simulink model "m1"  (R2020a)
settings: Solver=FixedStepAuto  StartTime=0.0  StopTime=25000.0  FixedStep=1  RelTol=1e-3
libraries: dspstat3 x12, simulink x2
settings Model: Creator=Kalev  LastModifiedBy=Kalev
settings OptimizationCC: ZeroExternalMemoryAtStartup=off  ZeroInternalMemoryAtStartup=off
settings HardwareCC: ProdBitPerPointer=32  ProdBitPerSizeT=32  ProdBitPerPtrDiffT=32  ProdLargestAtomicInteger=Long  ProdWordSize=32  ProdHWDeviceType=ARM Compatible->ARM 10
settings RTWCC: GenCodeOnly=on  TargetLang=C++
settings GRTTargetCC: TargetLangStandard=C++03 (ISO)  MultiInstanceERTCode=on  CodeInterfacePackaging=C++ class  RTWCAPIParams=on  RTWCAPIStates=on  MultiInstanceErrorCode=Warning

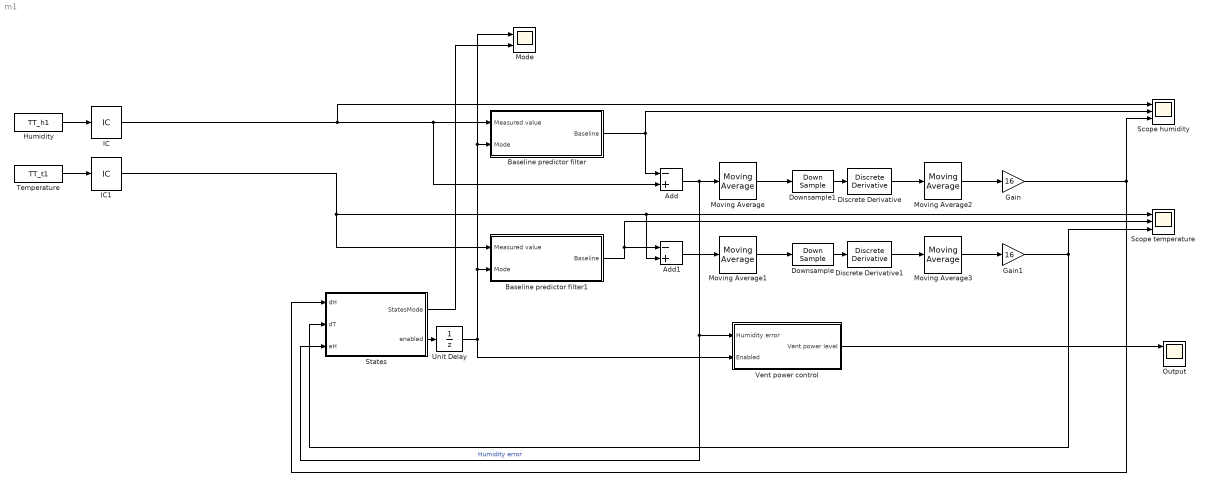
== system m1 ==
  Add : Sum  Inputs=-+
  Add1 : Sum  Inputs=-+
  Baseline predictor filter : Subsystem
  Baseline predictor filter1 : Subsystem
  Discrete Derivative : simulink/Discrete/Discrete Derivative  gainval=1.0  ICPrevScaledInput=initial_h  OutMin=[]  OutMax=[]  OutDataType=fixdt(1, 16)  OutScaling=2^-10  DoSatur=off
  Discrete Derivative1 : simulink/Discrete/Discrete Derivative  gainval=1.0  ICPrevScaledInput=initial_t  OutMin=[]  OutMax=[]  OutDataType=fixdt(1, 16)  OutScaling=2^-10  DoSatur=off
  Downsample : DownSample  N=16  phase=15  ic=initial_t
  Downsample1 : DownSample  N=16  phase=15  ic=initial_h
  Gain : Gain  Gain=16
  Gain1 : Gain  Gain=16
  Humidity : FromWorkspace  VariableName=TT_h1  OutDataTypeStr=double  SampleTime=-1
  IC : InitialCondition  Value=50
  IC1 : InitialCondition  Value=25
  Mode : Scope  NumInputPorts=2
  Moving Average{,1..3} (4 alike) : dspstat3/Moving Average  Method=Sliding window  ForgettingFactorPort=off  SpecifyWindowLength=on  WindowLength=16  ForgettingFactor=0.9  SimulateUsing=Code generation
  Output : Scope  NumInputPorts=3
  Scope humidity : Scope  NumInputPorts=3
  Scope temperature : Scope  NumInputPorts=3
  States : Stateflow chart  TreatAsAtomicUnit=on
  Temperature : FromWorkspace  VariableName=TT_t1  OutDataTypeStr=double  SampleTime=-1  OutputAfterFinalValue=Holding final value
  Unit Delay : UnitDelay  SampleTime=-1  HasFrameUpgradeWarning=on
  Vent power control : Subsystem
  wires:
  Humidity/1 -> IC/1
  Baseline predictor filter/1(Baseline) -> Scope humidity/2, Add/1
  Add/1 -> Vent power control/1(Humidity error), States/3(eH), Moving Average/1  "Humidity error"
  Temperature/1 -> IC1/1
  Add1/1 -> Moving Average1/1
  Discrete Derivative1/1 -> Moving Average3/1
  States/2(enabled) -> Unit Delay/1
  Unit Delay/1 -> Vent power control/2(Enabled), Baseline predictor filter1/2(Mode), Baseline predictor filter/2(Mode), Mode/1
  Downsample/1 -> Discrete Derivative1/1
  Downsample1/1 -> Discrete Derivative/1
  Baseline predictor filter1/1(Baseline) -> Add1/1, Scope temperature/2
  IC/1 -> Add/2, Baseline predictor filter/1(Measured value), Scope humidity/1
  IC1/1 -> Baseline predictor filter1/1(Measured value), Scope temperature/1, Add1/2
  Discrete Derivative/1 -> Moving Average2/1
  Moving Average/1 -> Downsample1/1
  Moving Average1/1 -> Downsample/1
  States/1(StatesMode) -> Mode/2
  Moving Average2/1 -> Gain/1
  Moving Average3/1 -> Gain1/1
  Gain/1 -> Scope humidity/3, States/1(dH)
  Gain1/1 -> Scope temperature/3, States/2(dT)
  Vent power control/1(Vent power level) -> Output/1

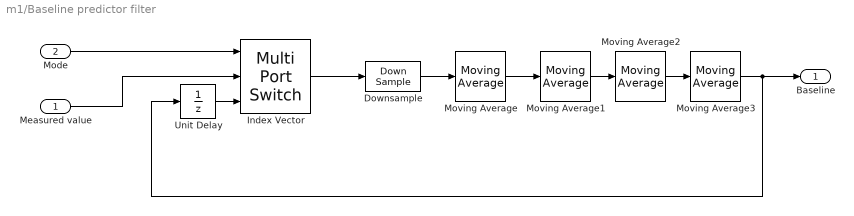
== system m1/Baseline predictor filter ==
  Measured value : Inport
  Mode : Inport  Port=2
  Downsample : DownSample  N=128
  Index Vector : MultiPortSwitch  DataPortOrder=Zero-based contiguous  Inputs=2  zeroidx=on
  Moving Average{,1..3} (4 alike) : dspstat3/Moving Average  Method=Sliding window  ForgettingFactorPort=off  SpecifyWindowLength=on  WindowLength=512  ForgettingFactor=0.9  SimulateUsing=Code generation
  Unit Delay : UnitDelay  SampleTime=-1  HasFrameUpgradeWarning=on
  Baseline : Outport
  wires:
  Moving Average1/1 -> Moving Average2/1
  Moving Average/1 -> Moving Average1/1
  Downsample/1 -> Moving Average/1
  Moving Average2/1 -> Moving Average3/1
  Index Vector/1 -> Downsample/1
  Mode/1 -> Index Vector/1
  Measured value/1 -> Index Vector/2
  Moving Average3/1 -> Unit Delay/1, Baseline/1
  Unit Delay/1 -> Index Vector/3

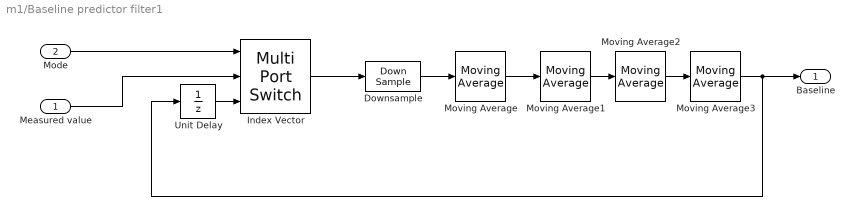
== system m1/Baseline predictor filter1 ==
  Measured value : Inport
  Mode : Inport  Port=2
  Downsample : DownSample  N=128
  Index Vector : MultiPortSwitch  DataPortOrder=Zero-based contiguous  Inputs=2  zeroidx=on
  Moving Average{,1..3} (4 alike) : dspstat3/Moving Average  Method=Sliding window  ForgettingFactorPort=off  SpecifyWindowLength=on  WindowLength=512  ForgettingFactor=0.9  SimulateUsing=Code generation
  Unit Delay : UnitDelay  SampleTime=-1  HasFrameUpgradeWarning=on
  Baseline : Outport
  wires:
  Unit Delay/1 -> Index Vector/3
  Index Vector/1 -> Downsample/1
  Moving Average3/1 -> Unit Delay/1, Baseline/1
  Measured value/1 -> Index Vector/2
  Mode/1 -> Index Vector/1
  Downsample/1 -> Moving Average/1
  Moving Average/1 -> Moving Average1/1
  Moving Average2/1 -> Moving Average3/1
  Moving Average1/1 -> Moving Average2/1

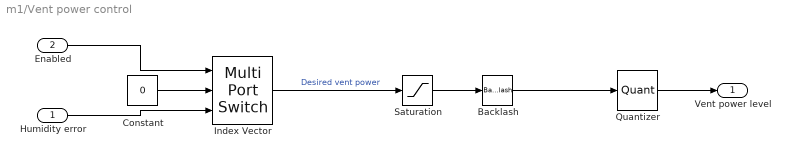
== system m1/Vent power control ==
  Humidity error : Inport
  Enabled : Inport  Port=2
  Backlash : Backlash  BacklashWidth=2
  Constant : Constant  Value=0
  Index Vector : MultiPortSwitch  DataPortOrder=Zero-based contiguous  Inputs=2  zeroidx=on
  Quantizer : Quantizer  QuantizationInterval=30/4  LinearizeAsGain=off
  Saturation : Saturate  UpperLimit=30  LowerLimit=0
  Vent power level : Outport
  wires:
  Constant/1 -> Index Vector/2
  Index Vector/1 -> Saturation/1  "Desired vent power"
  Humidity error/1 -> Index Vector/3
  Enabled/1 -> Index Vector/1
  Quantizer/1 -> Vent power level/1
  Saturation/1 -> Backlash/1
  Backlash/1 -> Quantizer/1

== stateflow chart m1/States ==
  state Stopping
    entry: enabled=0
  state Detected
    entry: enabled=1
  state Stable
    entry: enabled=1
  state OFF
    entry: enabled=0
  Stopping -> OFF
  Detected -> OFF [order 1] : [dH <  -5]
  Stable -> Stopping : [eH < 8]
  (default) -> OFF
  Detected -> Stable [order 2] : [eH > 10]
  OFF -> Detected : [dH > 4]
  data: dH input; dT input; StatesMode output Enum: StatesModeType; enabled output; eH input
